simulink model "poscontrol"  (R2020a)
settings: Solver=ode1  StartTime=0.0  StopTime=0.35  FixedStep=0.001  RelTol=1e-3  AbsTol=1e-6
PreLoadFcn:
  | if exist('tl_preloadfcn','file'), tl_preloadfcn(gcs,'5.2.0.24'); end
PostLoadFcn:
  | if exist('tl_postloadfcn','file'), tl_postloadfcn(gcs,'5.2.0.24'); end
InitFcn:
  | if exist('tlds_init','file'), tlds_init(gcs); end
StartFcn:
  | if exist('tlds_start','file'), tlds_start(gcs); end
StopFcn:
  | if exist('tlds_stop','file'), tlds_stop(gcs); end
values from neighbouring files (symbols this model uses):
  d = 0.5    [start.m]
  Ki = 0.2    [start.m]
  Kp = 2.0    (= 2)    [start.m]
  m = 0.01    [start.m]
  tab_in = [-12:12]'    [start.m]
  tab_out = max(tab_in)*tab_out/max(tab_out)    [start.m]
  tSample = 0.001    [start.m]
libraries: tllib x7
PreSaveFcn:
  | if exist('tl_presavefcn','file'), tl_presavefcn(gcs); end
CloseFcn:
  | if exist('tl_closefcn','file'), tl_closefcn(gcs); end
settings Model: Tag=0  DS_PROJECTFILE=poscontrol.dd  TL_MAIN_DATA={'codeopt',{'inliningthreshold',5,'assembler',1},'logopt',{'plotinterval',0.1},'date',738426.71050905087}  TL_MODEL_COMMENT=This demo model implements a PI controller with feedback linearization.  TLVersion=5.2.0.24  ExtModeTrigMode=oneshot  ExtModeArmWhenConnect=off  Creator=dSPACE GmbH  LastModifiedBy=dSPACE GmbH
settings SolverCC: AutoScaleAbsTol=off
settings DataIOCC: SaveFormat=Array  ReturnWorkspaceOutputs=off  SignalLoggingName=sigsOut
settings OptimizationCC: BlockReduction=off  BooleanDataType=off  OptimizeBlockIOStorage=off  BufferReuse=off  GlobalBufferReuse=off  ExpressionFolding=off  ExpressionDepthLimit=2147483647  LocalBlockOutputs=off  InitFltsAndDblsToZero=on  LifeSpan=inf  OptimizeDataStoreBuffers=off  BusAssignmentInplaceUpdate=off
settings DebuggingCC: SaveWithParameterizedLinksMsg=none  SignalResolutionControl=TryResolveAllWithWarning  MultiTaskDSMMsg=warning  MultiTaskCondExecSysMsg=none  FcnCallInpInsideContextMsg=warning  BusObjectLabelMismatch=error  StateNameClashWarn=warning  StrictBusMsg=ErrorOnBusTreatedAsVector  NonBusSignalsTreatedAsBus=error  SFUnexpectedBacktrackingDiag=warning  SFNoUnconditionalDefaultTransitionDiag=warning  SFExecutionAtInitializationDiag=none  ArithmeticOperatorsInVariantConditions=warning
settings HardwareCC: ProdBitPerPointer=32  ProdBitPerSizeT=32  ProdBitPerPtrDiffT=32  ProdLargestAtomicFloat=None  ProdIntDivRoundTo=Undefined  ProdEndianess=Unspecified  ProdWordSize=32  ProdHWDeviceType=32-bit Generic  TargetUnknown=on
settings ModelReferenceCC: PropagateSignalLabelsOutOfModel=off
settings SFSimCC: SimUseLocalCustomCode=off  CustomCodeUndefinedFunction=UseInterfaceOnly
settings RTWCC: TemplateMakefile=grt_vc.tmf  RTWUseLocalCustomCode=off
settings CodeAppCC: StateflowObjectComments=on
settings GRTTargetCC: TargetFcnLib=ansi_tfl_tmw.mat  TargetLangStandard=C89/C90 (ANSI)  ModelReferenceCompliant=off  CombineOutputUpdateFcns=off  MatFileLogging=off  GRTInterface=on
settings ConfigComp: CovMetricSettings=dw  CovHtmlReporting=on  CovSaveCumulativeToWorkspaceVar=on  CovSaveSingleToWorkspaceVar=on  CovExternalEMLEnable=off

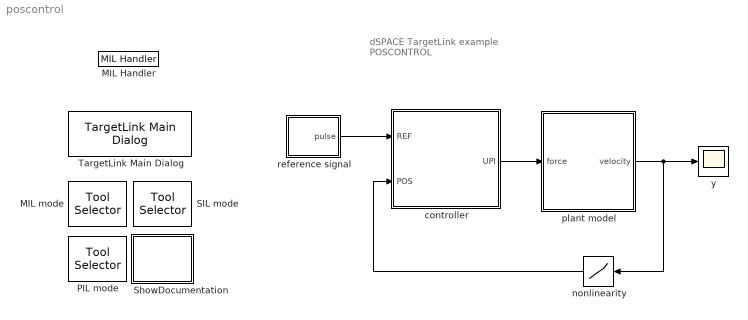
== system poscontrol ==
  note: dSPACE TargetLink example
      | POSCONTROL
  MIL Handler : tllib/MIL Handler  data={'date',738426.71051353007}
      settings: SourceProductName=dSPACE TargetLink common blockset
  MIL mode : tllib/Tool Selector  Description=MIL\nmode  data={'date',738426.710515243}
      settings: SourceProductName=dSPACE TargetLink common blockset
  PIL mode : tllib/Tool Selector  Description=PIL\nmode  data={'date',738426.71051530098}
      settings: SourceProductName=dSPACE TargetLink common blockset
  SIL mode : tllib/Tool Selector  Description=SIL\nmode  data={'date',738426.71051535883}
      settings: SourceProductName=dSPACE TargetLink common blockset
  ShowDocumentation : Subsystem
      settings: OpenFcn=if exist('tl_demos','file')==2,web([tl_get_specialfolder('TLInstallation'),'\Matlab\Demos\poscontrol\html\poscontrol.html']), end
      mask Display: disp('?')
  TargetLink Main Dialog : tllib/TargetLink Main Dialog  data=[]
      settings: SourceProductName=dSPACE TargetLink common blockset
  controller : Subsystem  Tag=TargetLink Simulation Frame  mask(TL_SimFrame){}
      settings: CopyFcn=if exist('tl_copyfcn','file'), tl_copyfcn(gcbh); end  NameChangeFcn=if exist('tl_framenamechangefcn','file'), tl_framenamechangefcn(gcbh); end
      settings: OpenFcn=|
      | if exist('open_tlsubsystem','file')
      |    open_tlsubsystem(gcbh);
      | else
      |    tlsubsystem = ...
      |       find_system(gcb, ...
      |       'LookUnderMasks','on', ...
      |       'FollowLinks','on', ...
      |       'Tag','MIL Subsystem');
      |    open_system(tlsubsystem);
      | end
      mask Display: disp('TargetLink\nModel-\nin-the-loop\nmode')
  nonlinearity : Lookup  InputValues=tab_in  Table=tab_out  SaturateOnIntegerOverflow=on
  plant model : Subsystem
  reference signal : Subsystem
  y : Scope
  wires:
  plant model/1(velocity) -> y/1, nonlinearity/1
  nonlinearity/1 -> controller/2(POS)
  controller/1(UPI) -> plant model/1(force)
  reference signal/1(pulse) -> controller/1(REF)

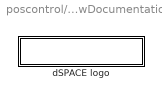
== system poscontrol/ShowDocumentation ==
  dSPACE logo : Subsystem
      mask Display: image(ds_get_icon('dspace_logo_bg_white_l'))

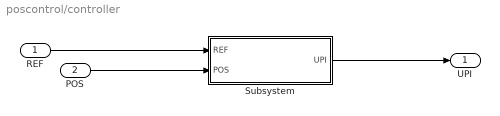
== system poscontrol/controller ==
  REF : Inport  SampleTime=tSample
  POS : Inport  Port=2  SampleTime=tSample
  Subsystem : Subsystem  Tag=struct('sfcnName','controller_sf','subFunction','','srcSubsystem','')  mask(TL_Enable){}
      settings: OpenFcn=warndlg(get_param(gcb,'MaskHelp'),'Serious Warning');
      mask Help: This subsystem keeps the TargetLink subsystem (subsystem with TargetLink blocks for production code generation), and is needed for the TargetLink simulation frame to work properly. DO NOT DELETE OR MODIFY IT!
  UPI : Outport  InitialOutput=0  VectorParamsAs1DForOutWhenUnconnected=off
  wires:
  REF/1 -> Subsystem/1(REF)
  POS/1 -> Subsystem/2(POS)
  Subsystem/1(UPI) -> UPI/1

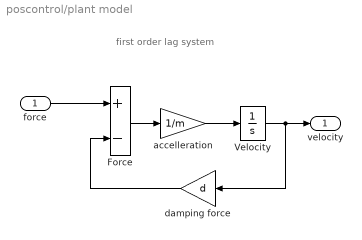
== system poscontrol/plant model ==
  note: first order lag system
  force : Inport
  Force : Sum  Inputs=+-  InputSameDT=on  SaturateOnIntegerOverflow=on  OutDataTypeStr=Inherit: Same as first input
  Velocity : Integrator
  accelleration : Gain  Gain=1/m  SaturateOnIntegerOverflow=on  OutDataTypeStr=Inherit: Same as input  ParamDataTypeStr=Inherit: Same as input
  damping force : Gain  Gain=d  SaturateOnIntegerOverflow=on  OutDataTypeStr=Inherit: Same as input  ParamDataTypeStr=Inherit: Same as input
  velocity : Outport  InitialOutput=0  VectorParamsAs1DForOutWhenUnconnected=off
  wires:
  Force/1 -> accelleration/1
  accelleration/1 -> Velocity/1
  force/1 -> Force/1
  Velocity/1 -> damping force/1, velocity/1
  damping force/1 -> Force/2

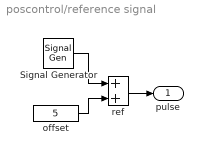
== system poscontrol/reference signal ==
  Signal Generator : SignalGenerator  WaveForm=square  Amplitude=5  Frequency=5
  offset : Constant  Value=5
  ref : Sum  InputSameDT=on  SaturateOnIntegerOverflow=on  OutDataTypeStr=Inherit: Same as first input
  pulse : Outport  InitialOutput=0  VectorParamsAs1DForOutWhenUnconnected=off
  wires:
  Signal Generator/1 -> ref/1
  offset/1 -> ref/2
  ref/1 -> pulse/1

== system poscontrol/ShowDocumentation/dSPACE logo ==

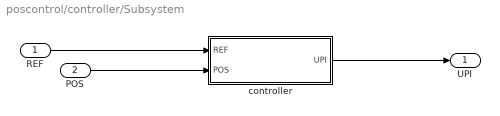
== system poscontrol/controller/Subsystem ==
  REF : Inport
  POS : Inport  Port=2
  controller : Subsystem  Tag=MIL Subsystem  Description=Ctrl  LoadFcn=|
      | if exist('TargetLink.SimFrameHandler.TLSubsystem','class')
      |     TargetLink.SimFrameHandler.TLSubsystem.CreateWatchDog(gcbh);
      | end
      settings: CopyFcn=if exist('tl_copyfcn','file'), tl_copyfcn(gcbh); end  NameChangeFcn=if exist('tl_namechangefcn','file'), tl_namechangefcn(gcbh); end  DestroyFcn=if exist('update_tl_main_dlg','file'), update_tl_main_dlg('TL_subs_display'); end
      mask Display: disp('TargetLink Subsystem')
  UPI : Outport  VectorParamsAs1DForOutWhenUnconnected=off
  wires:
  REF/1 -> controller/1(REF)
  POS/1 -> controller/2(POS)
  controller/1(UPI) -> UPI/1

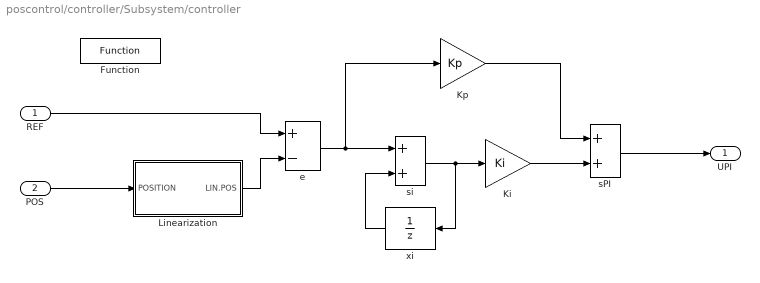
== system poscontrol/controller/Subsystem/controller ==
  REF : Inport  PortDimensions=1  SampleTime=tSample  mask(TL_Inport){data={'logdata',{'plotchannels',1},'output',{'variable','Reference'},'date',738426.71051222226}}
      settings: CopyFcn=if exist('copy_tlblock','file')==2,copy_tlblock(gcbh);end  DeleteFcn=if exist('delete_tlblock','file')==2,delete_tlblock(gcbh);end  NameChangeFcn=if exist('rename_tlblock','file')==2,rename_tlblock(gcbh);end  OpenFcn=if exist('tl_open_blockdlg','file')==2,tl_open_blockdlg(gcbh);else,open_system(gcbh,'force');end
      mask Help: eval(['if exist(''tl_online_help'',''file'') == 2, tl_online_help(''Topic'',''TL_Inport''),else, web([''jar:file:///'',matlabroot,''/help/toolbox/simulink/help.jar!/slref/' lower(get_param(gcbh,'Blocktype')) '.html''], ''-helpbrowser''),end'])
      mask Display:
      | [x,y] = tlDrawBrandOnBlockIcon(gcbh);
      | plot(x,y);
  POS : Inport  Port=2  PortDimensions=1  SampleTime=tSample  mask(TL_Inport){data={'logdata',{'plotchannels',1},'output',{'variable','Position'},'date',738426.71051254624}}
      settings: CopyFcn=if exist('copy_tlblock','file')==2,copy_tlblock(gcbh);end  DeleteFcn=if exist('delete_tlblock','file')==2,delete_tlblock(gcbh);end  NameChangeFcn=if exist('rename_tlblock','file')==2,rename_tlblock(gcbh);end  OpenFcn=if exist('tl_open_blockdlg','file')==2,tl_open_blockdlg(gcbh);else,open_system(gcbh,'force');end
      mask Help: eval(['if exist(''tl_online_help'',''file'') == 2, tl_online_help(''Topic'',''TL_Inport''),else, web([''jar:file:///'',matlabroot,''/help/toolbox/simulink/help.jar!/slref/' lower(get_param(gcbh,'Blocktype')) '.html''], ''-helpbrowser''),end'])
      mask Display:
      | [x,y] = tlDrawBrandOnBlockIcon(gcbh);
      | plot(x,y);
  Function : tllib/Function  data={'description',['controller function'],'stepfunctionname','Controller','restartfunctionname','RESTART_Controller','initfunctionname','INIT_Controller','termfunctionname','TERM_Controller','subsystemid','Ctrl','module','Controller','blockobject','ControllerSystem','signature','Controller','date',738426.71051069442}  displayString=FUNCTION
      settings: SourceProductName=dSPACE TargetLink common blockset
  Ki : Gain  Tag="Gain block of the dSPACE Fixed Point Code Generation Environment.      \\n                                                                       \\n signal is equal to the product of the input signal and the gain value:\\n\t\ty = G u"  Description=|  Gain=Ki  mask(TL_Gain){data={'logdata',{'plotchannels',1},'output',{'lsb',2^-9},'gain',{'name','P_$S_$B','type','UInt8','lsb',2^-8},'date',738426.71051127312}}
      | Gain block of dSPACE TargetLink.
      | 
      | Output signal is equal to the product of the input signal and the gain value:
      |         y = G u
      settings: CopyFcn=if exist('copy_tlblock','file')==2,copy_tlblock(gcbh);end  DeleteFcn=if exist('delete_tlblock','file')==2,delete_tlblock(gcbh);end  NameChangeFcn=if exist('rename_tlblock','file')==2,rename_tlblock(gcbh);end  OpenFcn=if exist('tl_open_blockdlg','file')==2,tl_open_blockdlg(gcbh);else,open_system(gcbh,'force');end
      mask Help: eval(['if exist(''tl_online_help'',''file'') == 2, tl_online_help(''Topic'',''TL_Gain''),else, web([''jar:file:///'',matlabroot,''/help/toolbox/simulink/help.jar!/slref/' lower(get_param(gcbh,'Blocktype')) '.html''], ''-helpbrowser''),end'])
      mask Display:
      | [x,y] = tlDrawBrandOnBlockIcon(gcbh);
      | plot(x,y);
  Kp : Gain  Description=|  Gain=Kp  mask(TL_Gain){data={'logdata',{'plotchannels',1},'output',{'lsb',2^-9},'gain',{'name','P_$S_$B','type','UInt8','lsb',2^-6},'date',738426.71051157406}}
      | Gain block of dSPACE TargetLink.
      | 
      | Output signal is equal to the product of the input signal and the gain value:
      |         y = G u
      settings: CopyFcn=if exist('copy_tlblock','file')==2,copy_tlblock(gcbh);end  DeleteFcn=if exist('delete_tlblock','file')==2,delete_tlblock(gcbh);end  NameChangeFcn=if exist('rename_tlblock','file')==2,rename_tlblock(gcbh);end  OpenFcn=if exist('tl_open_blockdlg','file')==2,tl_open_blockdlg(gcbh);else,open_system(gcbh,'force');end
      mask Help: eval(['if exist(''tl_online_help'',''file'') == 2, tl_online_help(''Topic'',''TL_Gain''),else, web([''jar:file:///'',matlabroot,''/help/toolbox/simulink/help.jar!/slref/' lower(get_param(gcbh,'Blocktype')) '.html''], ''-helpbrowser''),end'])
      mask Display:
      | [x,y] = tlDrawBrandOnBlockIcon(gcbh);
      | plot(x,y);
  Linearization : Subsystem  TreatAsAtomicUnit=on
  e : Sum  Description=|  Inputs=+-  mask(TL_Sum){data={'logdata',{'maxnumvals',4096,'plotchannels',1},'output',{'lsb',2^-10},'date',738426.71051450237}}
      | Sum block of dSPACE TargetLink.
      | 
      | Output signal is equal to the sum of the input signals.
      | The list of signs is specified according to conventions for Simulink Sum blocks.
      settings: CopyFcn=if exist('copy_tlblock','file')==2,copy_tlblock(gcbh);end  DeleteFcn=if exist('delete_tlblock','file')==2,delete_tlblock(gcbh);end  NameChangeFcn=if exist('rename_tlblock','file')==2,rename_tlblock(gcbh);end  OpenFcn=if exist('tl_open_blockdlg','file')==2,tl_open_blockdlg(gcbh);else,open_system(gcbh,'force');end
      mask Help: eval(['if exist(''tl_online_help'',''file'') == 2, tl_online_help(''Topic'',''TL_Sum''),else, web([''jar:file:///'',matlabroot,''/help/toolbox/simulink/help.jar!/slref/' lower(get_param(gcbh,'Blocktype')) '.html''], ''-helpbrowser''),end'])
      mask Display:
      | [x,y] = tlDrawBrandOnBlockIcon(gcbh);
      | plot(x,y);
  sPI : Sum  Tag="Sum block of the dSPACE Fixed Point Code Generation Environment.\\n                                                                \\nOutput signal is equal to the sum of the two input signals:     \\n                                                                \\n\t\ty = u1 - u2"  Description=|  mask(TL_Sum){data={'logdata',{'plotchannels',1},'output',{'variable','SPI'},'date',738426.71051469911}}
      | Sum block of dSPACE TargetLink.
      | 
      | Output signal is equal to the sum of the input signals.
      | The list of signs is specified according to conventions for Simulink Sum blocks.
      settings: CopyFcn=if exist('copy_tlblock','file')==2,copy_tlblock(gcbh);end  DeleteFcn=if exist('delete_tlblock','file')==2,delete_tlblock(gcbh);end  NameChangeFcn=if exist('rename_tlblock','file')==2,rename_tlblock(gcbh);end  OpenFcn=if exist('tl_open_blockdlg','file')==2,tl_open_blockdlg(gcbh);else,open_system(gcbh,'force');end
      mask Help: eval(['if exist(''tl_online_help'',''file'') == 2, tl_online_help(''Topic'',''TL_Sum''),else, web([''jar:file:///'',matlabroot,''/help/toolbox/simulink/help.jar!/slref/' lower(get_param(gcbh,'Blocktype')) '.html''], ''-helpbrowser''),end'])
      mask Display:
      | [x,y] = tlDrawBrandOnBlockIcon(gcbh);
      | plot(x,y);
  si : Sum  Tag="Sum block of the dSPACE Fixed Point Code Generation Environment.\\n                                                                \\nOutput signal is equal to the sum of the two input signals:     \\n                                                                \\n\t\ty = u1 - u2"  Description=|  mask(TL_Sum){data={'logdata',{'plotchannels',1},'output',{'lsb',2^-9},'date',738426.71051488421}}
      | Sum block of dSPACE TargetLink.
      | 
      | Output signal is equal to the sum of the input signals.
      | The list of signs is specified according to conventions for Simulink Sum blocks.
      settings: CopyFcn=if exist('copy_tlblock','file')==2,copy_tlblock(gcbh);end  DeleteFcn=if exist('delete_tlblock','file')==2,delete_tlblock(gcbh);end  NameChangeFcn=if exist('rename_tlblock','file')==2,rename_tlblock(gcbh);end  OpenFcn=if exist('tl_open_blockdlg','file')==2,tl_open_blockdlg(gcbh);else,open_system(gcbh,'force');end
      mask Help: eval(['if exist(''tl_online_help'',''file'') == 2, tl_online_help(''Topic'',''TL_Sum''),else, web([''jar:file:///'',matlabroot,''/help/toolbox/simulink/help.jar!/slref/' lower(get_param(gcbh,'Blocktype')) '.html''], ''-helpbrowser''),end'])
      mask Display:
      | [x,y] = tlDrawBrandOnBlockIcon(gcbh);
      | plot(x,y);
  xi : UnitDelay  Tag="Unit Delay block of the dSPACE Fixed Point Code Generation Environment.               \\n                                                                                      \\nOutput signal is equal to the input signal of the last sample step:                   \\n                                                                                      \\n\t\ty(k) = u(k-1).                                                                      \\n                                                                                      \\nIn the first sampling step, the output signal is initialized with 'initial condition':\\n                                                                                      \\n\t\ty(0) = initial condition"  Description=|  SampleTime=tSample  HasFrameUpgradeWarning=on  mask(TL_UnitDelay){data={'logdata',{'plotchannels',1},'output',{'lsb',2^-9},'state',{'lsb',2^-9},'date',738426.71051559027}}
      | Unit Delay block of dSPACE TargetLink.
      | 
      | Output signal is equal to the input signal of the last sample step:
      | 
      |         y(k) = u(k-1).
      | 
      | In the 1st sampling step, the output signal is initialized with 'initial condition':
      | 
      |         y(0) = initial condition
      settings: CopyFcn=if exist('copy_tlblock','file')==2,copy_tlblock(gcbh);end  DeleteFcn=if exist('delete_tlblock','file')==2,delete_tlblock(gcbh);end  NameChangeFcn=if exist('rename_tlblock','file')==2,rename_tlblock(gcbh);end  OpenFcn=if exist('tl_open_blockdlg','file')==2,tl_open_blockdlg(gcbh);else,open_system(gcbh,'force');end
      mask Help: eval(['if exist(''tl_online_help'',''file'') == 2, tl_online_help(''Topic'',''TL_UnitDelay''),else, web([''jar:file:///'',matlabroot,''/help/toolbox/simulink/help.jar!/slref/' lower(get_param(gcbh,'Blocktype')) '.html''], ''-helpbrowser''),end'])
      mask Display:
      | [x,y] = tlDrawBrandOnBlockIcon(gcbh);
      | plot(x,y);
  UPI : Outport  PortDimensions=1  InitialOutput=0  VectorParamsAs1DForOutWhenUnconnected=off  mask(TL_Outport){data={'logdata',{'maxnumvals',4096,'plotchannels',1,'loggingmode',1},'output',{'variable','UPI'},'date',738426.71051381947}}
      settings: CopyFcn=if exist('copy_tlblock','file')==2,copy_tlblock(gcbh);end  DeleteFcn=if exist('delete_tlblock','file')==2,delete_tlblock(gcbh);end  NameChangeFcn=if exist('rename_tlblock','file')==2,rename_tlblock(gcbh);end  OpenFcn=if exist('tl_open_blockdlg','file')==2,tl_open_blockdlg(gcbh);else,open_system(gcbh,'force');end
      mask Help: eval(['if exist(''tl_online_help'',''file'') == 2, tl_online_help(''Topic'',''TL_Outport''),else, web([''jar:file:///'',matlabroot,''/help/toolbox/simulink/help.jar!/slref/' lower(get_param(gcbh,'Blocktype')) '.html''], ''-helpbrowser''),end'])
      mask Display:
      | [x,y] = tlDrawBrandOnBlockIcon(gcbh);
      | plot(x,y);
  wires:
  sPI/1 -> UPI/1
  REF/1 -> e/1
  POS/1 -> Linearization/1(POSITION)
  Linearization/1(LIN.POS) -> e/2
  Kp/1 -> sPI/1
  Ki/1 -> sPI/2
  e/1 -> si/1, Kp/1
  xi/1 -> si/2
  si/1 -> xi/1, Ki/1

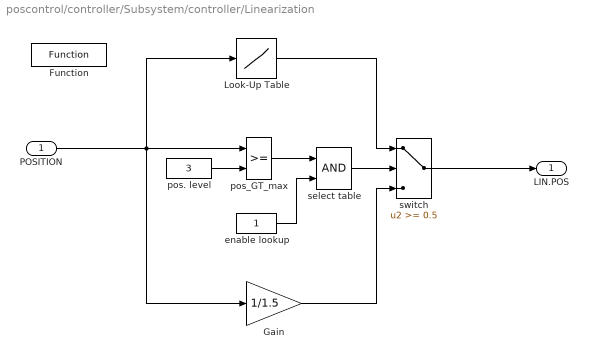
== system poscontrol/controller/Subsystem/controller/Linearization ==
  POSITION : Inport  PortDimensions=1  SampleTime=tSample  mask(TL_Inport){data={'logdata',{'plotchannels',1},'output',{'variable','Position'},'date',738426.71051284717}}
      settings: CopyFcn=if exist('copy_tlblock','file')==2,copy_tlblock(gcbh);end  DeleteFcn=if exist('delete_tlblock','file')==2,delete_tlblock(gcbh);end  NameChangeFcn=if exist('rename_tlblock','file')==2,rename_tlblock(gcbh);end  OpenFcn=if exist('tl_open_blockdlg','file')==2,tl_open_blockdlg(gcbh);else,open_system(gcbh,'force');end
      mask Help: eval(['if exist(''tl_online_help'',''file'') == 2, tl_online_help(''Topic'',''TL_Inport''),else, web([''jar:file:///'',matlabroot,''/help/toolbox/simulink/help.jar!/slref/' lower(get_param(gcbh,'Blocktype')) '.html''], ''-helpbrowser''),end'])
      mask Display:
      | [x,y] = tlDrawBrandOnBlockIcon(gcbh);
      | plot(x,y);
  Function : tllib/Function  data={'description',['Linearization of measured position signal'],'stepfunctionname','Linearization','restartfunctionname','RESTART_$D','initfunctionname','INIT_$D','termfunctionname','TERM_$D','codecomment',['Calculation of the liearized position'],'module','Controller','blockobject','LinearizationSystem','signature','Linearization','date',738426.71051096066}  displayString=FUNCTION
      settings: SourceProductName=dSPACE TargetLink common blockset
  Gain : Gain  Description=|  Gain=1/1.5  mask(TL_Gain){data={'logdata',{'plotchannels',1},'output',{'lsb',2^-10},'gain',{'variable','LinGain'},'date',738426.71051190968}}
      | Gain block of dSPACE TargetLink.
      | 
      | Output signal is equal to the product of the input signal and the gain value:
      |         y = G u
      settings: CopyFcn=if exist('copy_tlblock','file')==2,copy_tlblock(gcbh);end  DeleteFcn=if exist('delete_tlblock','file')==2,delete_tlblock(gcbh);end  NameChangeFcn=if exist('rename_tlblock','file')==2,rename_tlblock(gcbh);end  OpenFcn=if exist('tl_open_blockdlg','file')==2,tl_open_blockdlg(gcbh);else,open_system(gcbh,'force');end
      mask Help: eval(['if exist(''tl_online_help'',''file'') == 2, tl_online_help(''Topic'',''TL_Gain''),else, web([''jar:file:///'',matlabroot,''/help/toolbox/simulink/help.jar!/slref/' lower(get_param(gcbh,'Blocktype')) '.html''], ''-helpbrowser''),end'])
      mask Display:
      | [x,y] = tlDrawBrandOnBlockIcon(gcbh);
      | plot(x,y);
  Look-Up Table : Lookup_n-D  Description=|  NumberOfTableDimensions=1  BreakpointsForDimension1=tab_in  BreakpointsForDimension2=[1:3]  IndexSearchMethod=Evenly spaced points  Table=tab_out  ExtrapMethod=Clip  InputSameDT=on  mask(TL_Lookup1D){data={'logdata',{'maxnumvals',4096,'plotchannels',1},'input',{'description',['measured position values'],'max',12,'min',-12,'lsb',2^-3,'unit','mm','x0',-12,'xn',12},'output',{'type','Int8','lsb',2^-3},'table',{'variable','LinTable'},'generatemapstruct',0,'date',738426.71051337966}}
      | Look-up table of dSPACE TargetLink.
      | 
      | This block calculates the output values dependant on the given characteristic. Note that the vector of input values must be monotonically increasing for TargetLink.
      settings: CopyFcn=if exist('copy_tlblock','file')==2,copy_tlblock(gcbh);end  DeleteFcn=if exist('delete_tlblock','file')==2,delete_tlblock(gcbh);end  NameChangeFcn=if exist('rename_tlblock','file')==2,rename_tlblock(gcbh);end  OpenFcn=if exist('tl_open_blockdlg','file')==2,tl_open_blockdlg(gcbh);else,open_system(gcbh,'force');end
      mask Help: eval(['if exist(''tl_online_help'',''file'') == 2, tl_online_help(''Topic'',''TL_Lookup1D''),else, web([''jar:file:///'',matlabroot,''/help/toolbox/simulink/help.jar!/slref/' lower(get_param(gcbh,'Blocktype')) '.html''], ''-helpbrowser''),end'])
      mask Display:
      | [x,y] = tlDrawBrandOnBlockIcon(gcbh);
      | plot(x,y);
  enable lookup : Constant  Tag=Constant block of the dSPACE Fixed Point Code Generation Environment.\n\nOutput signal keeps the given constant value.  Description=|  mask(TL_Constant){data={'output',{'variable','LinEnableLUT'},'date',738426.71051027777}}
      | Constant block of dSPACE TargetLink.
      | 
      | Output signal keeps the given constant value.
      settings: CopyFcn=if exist('copy_tlblock','file')==2,copy_tlblock(gcbh);end  DeleteFcn=if exist('delete_tlblock','file')==2,delete_tlblock(gcbh);end  NameChangeFcn=if exist('rename_tlblock','file')==2,rename_tlblock(gcbh);end  OpenFcn=if exist('tl_open_blockdlg','file')==2,tl_open_blockdlg(gcbh);else,open_system(gcbh,'force');end
      mask Help: eval(['if exist(''tl_online_help'',''file'') == 2, tl_online_help(''Topic'',''TL_Constant''),else, web([''jar:file:///'',matlabroot,''/help/toolbox/simulink/help.jar!/slref/' lower(get_param(gcbh,'Blocktype')) '.html''], ''-helpbrowser''),end'])
      mask Display:
      | [x,y] = tlDrawBrandOnBlockIcon(gcbh);
      | plot(x,y);
  pos. level : Constant  Description=|  Value=3  mask(TL_Constant){data={'output',{'lsb',2^-10},'date',738426.71051047451}}
      | Constant block of dSPACE TargetLink.
      | 
      | Output signal keeps the given constant value.
      settings: CopyFcn=if exist('copy_tlblock','file')==2,copy_tlblock(gcbh);end  DeleteFcn=if exist('delete_tlblock','file')==2,delete_tlblock(gcbh);end  NameChangeFcn=if exist('rename_tlblock','file')==2,rename_tlblock(gcbh);end  OpenFcn=if exist('tl_open_blockdlg','file')==2,tl_open_blockdlg(gcbh);else,open_system(gcbh,'force');end
      mask Help: eval(['if exist(''tl_online_help'',''file'') == 2, tl_online_help(''Topic'',''TL_Constant''),else, web([''jar:file:///'',matlabroot,''/help/toolbox/simulink/help.jar!/slref/' lower(get_param(gcbh,'Blocktype')) '.html''], ''-helpbrowser''),end'])
      mask Display:
      | [x,y] = tlDrawBrandOnBlockIcon(gcbh);
      | plot(x,y);
  pos_GT_max : RelationalOperator  Description=|  RndMeth=Nearest  mask(TL_RelationalOperator){data={'date',738426.71051431715}}
      | Relational operator block of dSPACE TargetLink.
      | 
      | This block performs a relational operation on its two inputs u1 and u2 and produces output according to the following table.
      | If the result is TRUE, the output is 1; if FALSE, it is 0.
      | 
      | Operator   Output
      |  ==        TRUE if u1 is equal to u2
      |  !=        TRUE if u1 is not equal to u2
      |  <         TRUE if u1 is less than u2
      |  <=        TRUE if u1 is less than or equal to u2
      |  >=        TRUE if u1 is greater than or equal to u2
      |  >         TRUE if u1 is greater than u2
      settings: CopyFcn=if exist('copy_tlblock','file')==2,copy_tlblock(gcbh);end  DeleteFcn=if exist('delete_tlblock','file')==2,delete_tlblock(gcbh);end  NameChangeFcn=if exist('rename_tlblock','file')==2,rename_tlblock(gcbh);end  OpenFcn=if exist('tl_open_blockdlg','file')==2,tl_open_blockdlg(gcbh);else,open_system(gcbh,'force');end
      mask Help: eval(['if exist(''tl_online_help'',''file'') == 2, tl_online_help(''Topic'',''TL_RelationalOperator''),else, web([''jar:file:///'',matlabroot,''/help/toolbox/simulink/help.jar!/slref/' lower(get_param(gcbh,'Blocktype')) '.html''], ''-helpbrowser''),end'])
      mask Display:
      | [x,y] = tlDrawBrandOnBlockIcon(gcbh);
      | plot(x,y);
  select table : Logic  Description=|  AllPortsSameDT=off  mask(TL_LogicalOperator){data={'date',738426.71051303239}}
      | Logical operator block of dSPACE TargetLink.
      | 
      | The Logical Operator block performs any of these logical operations on its inputs: AND, OR, NAND, NOR, XOR, and NOT. A nonzero input is treated as TRUE (1), a zero input as FALSE (0). The output depends on the selected operator. The output is 1 if TRUE and 0 if FALSE.
      settings: CopyFcn=if exist('copy_tlblock','file')==2,copy_tlblock(gcbh);end  DeleteFcn=if exist('delete_tlblock','file')==2,delete_tlblock(gcbh);end  NameChangeFcn=if exist('rename_tlblock','file')==2,rename_tlblock(gcbh);end  OpenFcn=if exist('tl_open_blockdlg','file')==2,tl_open_blockdlg(gcbh);else,open_system(gcbh,'force');end
      mask Help: eval(['if exist(''tl_online_help'',''file'') == 2, tl_online_help(''Topic'',''TL_LogicalOperator''),else, web([''jar:file:///'',matlabroot,''/help/toolbox/simulink/help.jar!/slref/' lower(get_param(gcbh,'Blocktype')) '.html''], ''-helpbrowser''),end'])
      mask Display:
      | [x,y] = tlDrawBrandOnBlockIcon(gcbh);
      | plot(x,y);
  switch : Switch  Description=|  Threshold=0.5  mask(TL_Switch){data={'logdata',{'maxnumvals',4096,'plotchannels',1},'output',{'lsb',2^-10},'threshold',{'name','P_$S_$B'},'date',738426.71051512728}}
      | Switch block of dSPACE TargetLink.
      | 
      | Passes through input 1 if input 2 is greater than or equal to threshold, otherwise, passes through input 3:
      | 
      | if u2 >= threshold
      |    y = u1;
      | else
      |    y = u3;
      | end
      settings: CopyFcn=if exist('copy_tlblock','file')==2,copy_tlblock(gcbh);end  DeleteFcn=if exist('delete_tlblock','file')==2,delete_tlblock(gcbh);end  NameChangeFcn=if exist('rename_tlblock','file')==2,rename_tlblock(gcbh);end  OpenFcn=if exist('tl_open_blockdlg','file')==2,tl_open_blockdlg(gcbh);else,open_system(gcbh,'force');end
      mask Help: eval(['if exist(''tl_online_help'',''file'') == 2, tl_online_help(''Topic'',''TL_Switch''),else, web([''jar:file:///'',matlabroot,''/help/toolbox/simulink/help.jar!/slref/' lower(get_param(gcbh,'Blocktype')) '.html''], ''-helpbrowser''),end'])
      mask Display:
      | [x,y] = tlDrawBrandOnBlockIcon(gcbh);
      | plot(x,y);
  LIN.POS : Outport  PortDimensions=1  InitialOutput=0  VectorParamsAs1DForOutWhenUnconnected=off  mask(TL_Outport){data={'logdata',{'maxnumvals',4096,'plotchannels',1,'loggingmode',1},'output',{'variable','LinPosition'},'date',738426.71051413193}}
      settings: CopyFcn=if exist('copy_tlblock','file')==2,copy_tlblock(gcbh);end  DeleteFcn=if exist('delete_tlblock','file')==2,delete_tlblock(gcbh);end  NameChangeFcn=if exist('rename_tlblock','file')==2,rename_tlblock(gcbh);end  OpenFcn=if exist('tl_open_blockdlg','file')==2,tl_open_blockdlg(gcbh);else,open_system(gcbh,'force');end
      mask Help: eval(['if exist(''tl_online_help'',''file'') == 2, tl_online_help(''Topic'',''TL_Outport''),else, web([''jar:file:///'',matlabroot,''/help/toolbox/simulink/help.jar!/slref/' lower(get_param(gcbh,'Blocktype')) '.html''], ''-helpbrowser''),end'])
      mask Display:
      | [x,y] = tlDrawBrandOnBlockIcon(gcbh);
      | plot(x,y);
  wires:
  Look-Up Table/1 -> switch/1
  pos. level/1 -> pos_GT_max/2
  enable lookup/1 -> select table/2
  Gain/1 -> switch/3
  select table/1 -> switch/2
  pos_GT_max/1 -> select table/1
  POSITION/1 -> pos_GT_max/1, Gain/1, Look-Up Table/1
  switch/1 -> LIN.POS/1
